simulink model "motoreCCsim"  (R2020b)
settings: Solver=VariableStepAuto  StartTime=0.0  StopTime=10.0  RelTol=1e-3
undefined symbols (not defined in the file or in its folder): kt, Rm
settings Model: Creator=marco  LastModifiedBy=marco

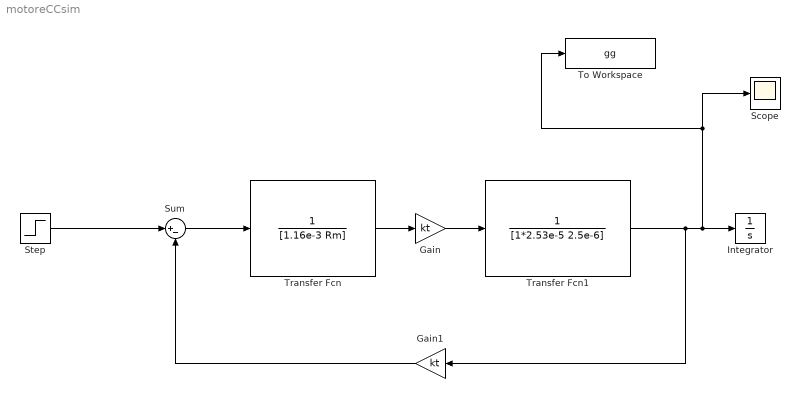
== system motoreCCsim ==
  Gain : Gain  Gain=kt
  Gain1 : Gain  Gain=kt
  Integrator : Integrator
  Scope : Scope
  Step : Step  Time=3  Before=2  After=4  SampleTime=0
  Sum : Sum  Inputs=|+-
  To Workspace : ToWorkspace  VariableName=gg  SaveFormat=Structure With Time  SampleTime=-1
  Transfer Fcn : TransferFcn  Denominator=[1.16e-3 Rm]
  Transfer Fcn1 : TransferFcn  Denominator=[1*2.53e-5 2.5e-6]
  wires:
  Gain/1 -> Transfer Fcn1/1
  Transfer Fcn1/1 -> Gain1/1, To Workspace/1, Scope/1, Integrator/1
  Transfer Fcn/1 -> Gain/1
  Sum/1 -> Transfer Fcn/1
  Gain1/1 -> Sum/2
  Step/1 -> Sum/1
